simulink model "switch_real_test"  (R2020a)
settings: Solver=VariableStepAuto  StartTime=0.0  StopTime=50  RelTol=1e-3
undefined symbols (not defined in the file or in its folder): Ap, Bp, Cp, Dp
libraries: simulink x2
settings Model: Creator=kekatos  LastModifiedBy=kekatos

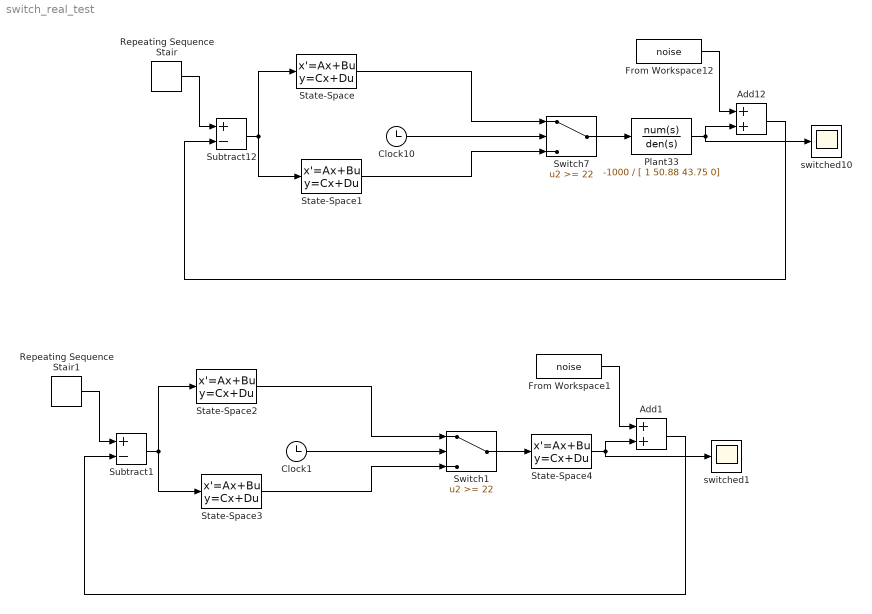
== system switch_real_test ==
  Add1 : Sum
  Add12 : Sum
  Clock1 : Clock
  Clock10 : Clock
  From Workspace1 : FromWorkspace  VariableName=noise
  From Workspace12 : FromWorkspace  VariableName=noise
  Plant33 : TransferFcn  Numerator=-1000  Denominator=[ 1 50.88 43.75 0]
  Repeating Sequence Stair : simulink/Sources/Repeating Sequence Stair  OutValues=[1 1 1 1 1 0 0 0 0 0].'  tsamp=2  OutMin=[]  OutMax=[]  OutDataTypeStr=double  OutputDataTypeScalingMode=double  OutDataType=fixdt(0,8)  ConRadixGroup=Best Precision: Vector-wise  OutScaling=2^-12
  Repeating Sequence Stair1 : simulink/Sources/Repeating Sequence Stair  OutValues=[1 1 1 1 1 0 0 0 0 0].'  tsamp=2  OutMin=[]  OutMax=[]  OutDataTypeStr=double  OutputDataTypeScalingMode=double  OutDataType=fixdt(0,8)  ConRadixGroup=Best Precision: Vector-wise  OutScaling=2^-12
  State-Space : StateSpace  A=[-63.28 -23.49 -8.735 ; 32 0 0;0 16 0]  B=[ 4 0 0]'  C=[-1.673 -2.665 -0.1544]  D=0  InitialCondition=0
  State-Space1 : StateSpace  A=[-974.2 -924.3 -457.2;512 0 0;0 512 0]  B=[2048; 0; 0]  C=[-2335 -306.9 -0.5891]  D=0  InitialCondition=0
  State-Space2 : StateSpace  A=[-63.28 -23.49 -8.735 ; 32 0 0;0 16 0]  B=[ 4 0 0]'  C=[-1.673 -2.665 -0.1544]  D=0  InitialCondition=0
  State-Space3 : StateSpace  A=[-974.2 -924.3 -457.2;512 0 0;0 512 0]  B=[2048; 0; 0]  C=[-2335 -306.9 -0.5891]  D=0  InitialCondition=0
  State-Space4 : StateSpace  A=Ap  B=Bp  C=Cp  D=Dp  InitialCondition=0
  Subtract1 : Sum  Inputs=+-
  Subtract12 : Sum  Inputs=+-
  Switch1 : Switch  Threshold=22
  Switch7 : Switch  Threshold=22
  switched1 : Scope
  switched10 : Scope
  wires:
  State-Space1/1 -> Switch7/3
  Plant33/1 -> Add12/2, switched10/1
  Switch7/1 -> Plant33/1
  Clock10/1 -> Switch7/2
  Subtract12/1 -> State-Space/1, State-Space1/1
  Add12/1 -> Subtract12/2
  State-Space/1 -> Switch7/1
  From Workspace12/1 -> Add12/1
  Repeating Sequence Stair/1 -> Subtract12/1
  Clock1/1 -> Switch1/2
  From Workspace1/1 -> Add1/1
  Subtract1/1 -> State-Space2/1, State-Space3/1
  Add1/1 -> Subtract1/2
  State-Space2/1 -> Switch1/1
  Switch1/1 -> State-Space4/1
  Repeating Sequence Stair1/1 -> Subtract1/1
  State-Space4/1 -> Add1/2, switched1/1
  State-Space3/1 -> Switch1/3
